simulink model "Model_2b"  (R2015b)
settings: Solver=ode45  StartTime=0.0  StopTime=25  RelTol=1e-3
undefined symbols (not defined in the file): a, b, c, d, K1, p1, Ts
settings Model: Creator=s3blanch  LastModifiedBy=s3blanch
settings DataIOCC: SaveFormat=StructureWithTime
settings HardwareCC: ProdWordSize=32  ProdHWDeviceType=Specified

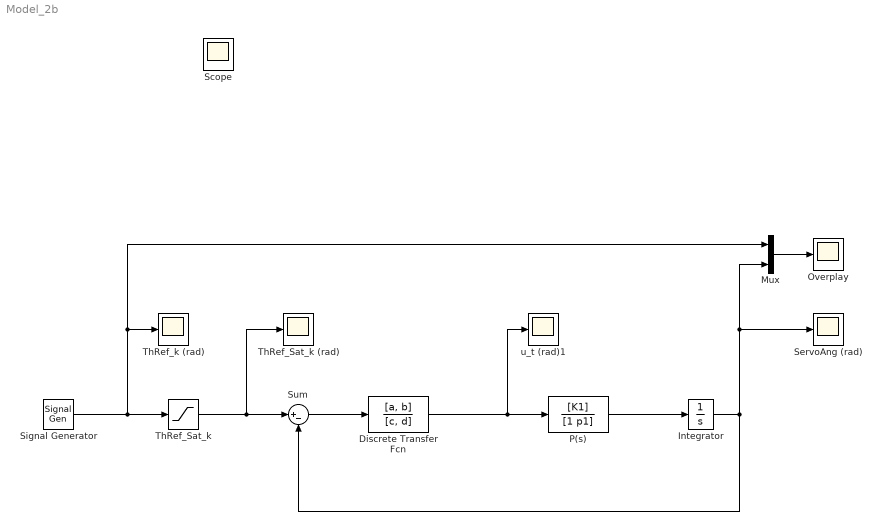
== system Model_2b ==
  Discrete Transfer Fcn : DiscreteTransferFcn  Numerator=[a, b]  Denominator=[c, d]  SampleTime=Ts
  Integrator : Integrator
  Mux : Mux  Inputs=2
  Overplay : Scope
  P(s) : TransferFcn  Numerator=[K1]  Denominator=[1 p1]
  ServoAng (rad) : Scope
  Signal Generator : SignalGenerator  WaveForm=square  Amplitude=0.5  Units=rad/sec
  Sum : Sum  Inputs=|+-
  ThRef_Sat_k : Saturate  UpperLimit=0.7  LowerLimit=-0.7
  ThRef_Sat_k (rad) : Scope
  ThRef_k (rad) : Scope
  u_t (rad)1 : Scope
  Scope : Scope
  wires:
  P(s)/1 -> Integrator/1
  Integrator/1 -> Mux/2, ServoAng (rad)/1, Sum/2
  Mux/1 -> Overplay/1
  ThRef_Sat_k/1 -> Sum/1, ThRef_Sat_k (rad)/1
  Signal Generator/1 -> Mux/1, ThRef_k (rad)/1, ThRef_Sat_k/1
  Sum/1 -> Discrete Transfer Fcn/1
  Discrete Transfer Fcn/1 -> u_t (rad)1/1, P(s)/1
